simulink model "FinalSimulink"  (R2021b)
settings: Solver=VariableStepAuto  StartTime=0.0  StopTime=10.0  RelTol=1e-3
settings Model: Creator=rkhas  LastModifiedBy=rkhas

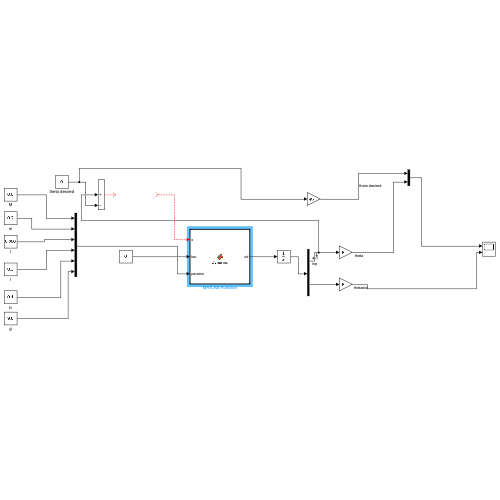
[thumbnail: Simulink's stored preview of the top-level diagram]
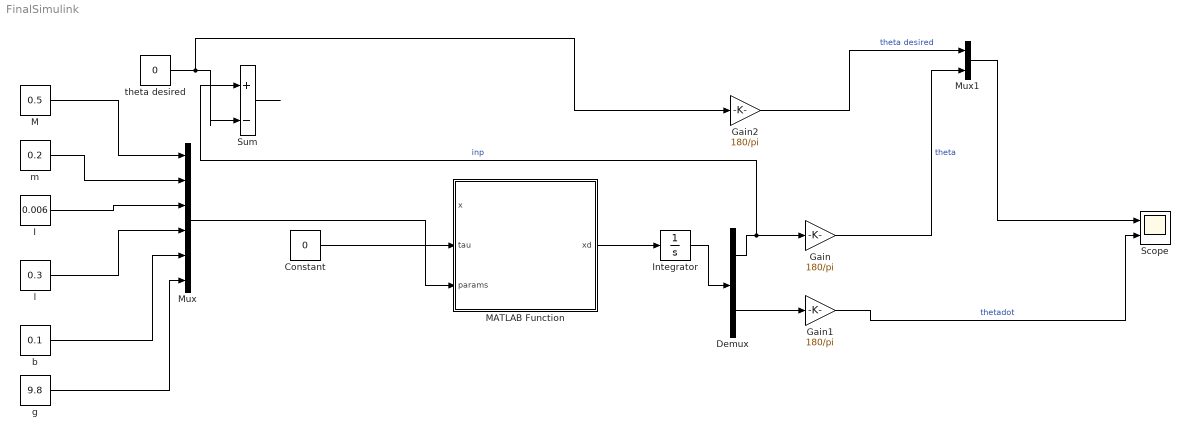
== system FinalSimulink ==
  Constant : Constant  Value=0
  Demux : Demux  Outputs=2
  Gain : Gain  Gain=180/pi
  Gain1 : Gain  Gain=180/pi
  Gain2 : Gain  Gain=180/pi
  I : Constant  Value=0.006
  Integrator : Integrator  InitialCondition=pi/2
  M : Constant  Value=0.5
  MATLAB Function : MATLAB Function  TreatAsAtomicUnit=on
  Mux : Mux  Inputs=6
  Mux1 : Mux  Inputs=2
  Scope : Scope  NumInputPorts=2
  Sum : Sum  Inputs=|+-
  b : Constant  Value=0.1
  g : Constant  Value=9.8
  l : Constant  Value=0.3
  m : Constant  Value=0.2
  theta desired : Constant  Value=0
  wires:
  Integrator/1 -> Demux/1
  Gain/1 -> Mux1/2  "theta"
  Demux/1 -> Sum/1, Gain/1  "inp"
  Sum/1 -> ?
  g/1 -> Mux/6
  Demux/2 -> Gain1/1
  Gain1/1 -> Scope/2  "thetadot"
  I/1 -> Mux/3
  l/1 -> Mux/4
  Mux/1 -> MATLAB Function/3(params)
  Mux1/1 -> Scope/1
  m/1 -> Mux/2
  Gain2/1 -> Mux1/1  "theta desired"
  b/1 -> Mux/5
  M/1 -> Mux/1
  MATLAB Function/1(xd) -> Integrator/1
  theta desired/1 -> Gain2/1, Sum/2
  ? -> MATLAB Function/1(x)
  Constant/1 -> MATLAB Function/2(tau)

== matlab function FinalSimulink/MATLAB Function ==
  data: x input; tau input; xd output; params input
function xd = Dynamic(x,tau,params)
M = params(1);
m = params(2);
b = params(5);
I = params(3);
g = params(6);
l = params(4);
Sy = sin(x(1));
Cy = cos(x(1));
D = m*l*l*(M+m*(1-Cy^2));
xd=zeros(2,1);
xd(1,1) = x(1);
xd(2,1) = (1/D)*((m+M)*m*g*l*Sy - m*l*Cy*(m*l*tau^2*Sy)) ;
xd=[xd(1,1);xd(2,1)];
